simulink model "control_simLEAD"  (R2024b)
settings: Solver=ode4  StartTime=0.0  StopTime=10  FixedStep=0.001  RelTol=1e-3
settings Model: Creator=henri  LastModifiedBy=henri

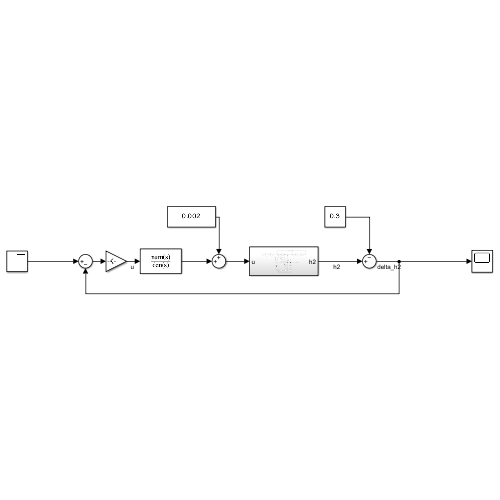
[thumbnail: Simulink's stored preview of the top-level diagram]
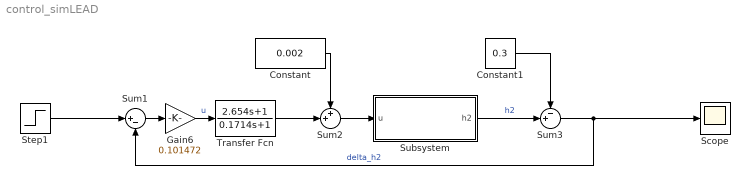
== system control_simLEAD ==
  Constant : Constant  Value=0.002
  Constant1 : Constant  Value=0.3
  Gain6 : Gain  Gain=0.101472
  Scope : Scope
  Step1 : Step  SampleTime=0
  Subsystem : Subsystem
  Sum1 : Sum  Inputs=|+-
  Sum2 : Sum  Inputs=++|
  Sum3 : Sum  Inputs=-+|
  Transfer Fcn : TransferFcn  Numerator=[2.654 1]  Denominator=[0.1714 1]
  wires:
  Sum1/1 -> Gain6/1
  Sum3/1 -> Sum1/2, Scope/1  "delta_h2"
  Sum2/1 -> Subsystem/1(u)
  Constant1/1 -> Sum3/1
  Subsystem/1(h2) -> Sum3/2  "h2"
  Step1/1 -> Sum1/1
  Constant/1 -> Sum2/1
  Gain6/1 -> Transfer Fcn/1  "u"
  Transfer Fcn/1 -> Sum2/2

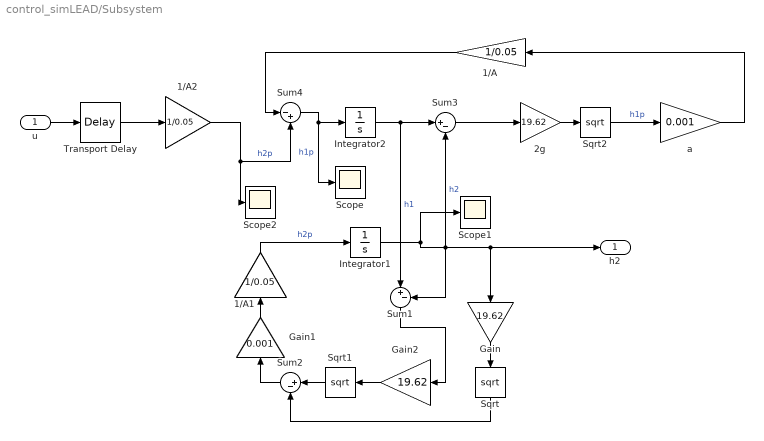
== system control_simLEAD/Subsystem ==
  u : Inport
  1/A : Gain  Gain=1/0.05
  1/A1 : Gain  Gain=1/0.05
  1/A2 : Gain  Gain=1/0.05
  2g : Gain  Gain=19.62
  Gain : Gain  Gain=19.62
  Gain1 : Gain  Gain=0.001
  Gain2 : Gain  Gain=19.62
  Integrator1 : Integrator  InitialCondition=0.3
  Integrator2 : Integrator  InitialCondition=0.6
  Scope : Scope
  Scope1 : Scope
  Scope2 : Scope
  Sqrt : Sqrt
  Sqrt1 : Sqrt
  Sqrt2 : Sqrt
  Sum1 : Sum  Inputs=|+-
  Sum2 : Sum  Inputs=|+-
  Sum3 : Sum  Inputs=|+-
  Sum4 : Sum  Inputs=|-+
  Transport Delay : TransportDelay  DelayTime=0
  a : Gain  Gain=0.001
  h2 : Outport
  wires:
  Sqrt/1 -> Sum2/2
  Sum3/1 -> 2g/1
  2g/1 -> Sqrt2/1
  Gain2/1 -> Sqrt1/1
  Gain/1 -> Sqrt/1
  Integrator1/1 -> Sum3/2, h2/1, Gain/1, Sum1/2, Scope1/1  "h2"
  Integrator2/1 -> Sum3/1, Sum1/1  "h1"
  Sum2/1 -> Gain1/1
  Sqrt1/1 -> Sum2/1
  Sqrt2/1 -> a/1  "h1p"
  Sum1/1 -> Gain2/1
  u/1 -> Transport Delay/1
  a/1 -> 1/A/1
  Sum4/1 -> Scope/1, Integrator2/1  "h1p"
  1/A/1 -> Sum4/1
  1/A1/1 -> Integrator1/1  "h2p"
  Gain1/1 -> 1/A1/1
  Transport Delay/1 -> 1/A2/1
  1/A2/1 -> Scope2/1, Sum4/2  "h2p"
